simulink model "CHM2Ctrl_Caller"  (R2018b)
settings: Solver=FixedStepDiscrete  StartTime=0.0  StopTime=10.0  FixedStep=0.01  RelTol=1e-3
undefined symbols (not defined in the file or in its folder): CHM2ActiveReqChk_Cal, CHM2ActiveSubStateCtrl_Cal, CHM2StateCtrl_Cal, KeSMSbMdChime2Enable_Val
settings Model: Creator=sn2xws  LastModifiedBy=sn2xws
settings DataIOCC: SaveFormat=StructureWithTime
settings OptimizationCC: DefaultParameterBehavior=Inlined  EnhancedBackFolding=on  PassReuseOutputArgsAs=Individual arguments  ZeroExternalMemoryAtStartup=off  ZeroInternalMemoryAtStartup=off  OptimizeBlockOrder=speed  DifferentSizesBufferReuse=on  OptimizationCustomize=off
settings DebuggingCC: ParameterTunabilityLossMsg=error
settings SFSimCC: MATLABDynamicMemAlloc=off
settings RTWCC: SystemTargetFile=autosar.tlc  GenCodeOnly=on  TemplateMakefile=ert_default_tmf  Description=AUTOSAR  GenerateReport=on  IncludeHyperlinkInReport=on  LaunchReport=on  GenerateTraceInfo=on  GenerateTraceReport=on  GenerateTraceReportSl=on  GenerateTraceReportSf=on  GenerateTraceReportEml=on  GenerateCodeMetricsReport=on
settings CodeAppCC: ForceParamTrailComments=on  IgnoreCustomStorageClasses=off  OperatorAnnotations=on  SimulinkDataObjDesc=on  SFDataObjDesc=on  InsertBlockDesc=on
settings STFCustomTargetCC: TargetLangStandard=C99 (ISO)  MultiwordLength=256  ParMdlRefBuildCompliant=on  CompOptLevelCompliant=on  IncludeMdlTerminateFcn=off  CombineOutputUpdateFcns=on  SuppressErrorStatus=on  ERTCustomFileBanners=on  SupportNonFinite=off  SupportComplex=off  SupportContinuousTime=off  SupportNonInlinedSFcns=off  RemoveResetFunc=on  MATLABClassNameForMDSCustomization=Simulink.SoftwareTarget.ERTCustomization  AutosarCompliant=on  UseToolchainInfoCompliant=on  LookupTableObjectStructAxisOrder=2,1,3,4,...  LUTObjectStructOrderEvenSpacing=Size,Table,Breakpoints  SystemTargetFile=autosar.tlc
settings ERTTargetCC: TargetLangStandard=C99 (ISO)  ConcurrentExecutionCompliant=off  IncludeMdlTerminateFcn=off  SuppressErrorStatus=on  SupportNonFinite=off  SupportComplex=off  ModelStepFunctionPrototypeControlCompliant=off  CPPClassGenCompliant=off  AutosarCompliant=on  LookupTableObjectStructAxisOrder=2,1,3,4,...  LUTObjectStructOrderEvenSpacing=Size,Table,Breakpoints  InlinedParameterPlacement=NonHierarchical  ERTCustomFileTemplate=example_file_process.tlc  ERTFilePackagingFormat=Compact

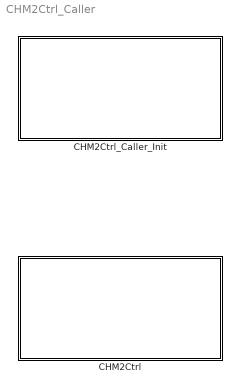
== system CHM2Ctrl_Caller ==
  CHM2Ctrl : Subsystem
  CHM2Ctrl_Caller_Init : Subsystem

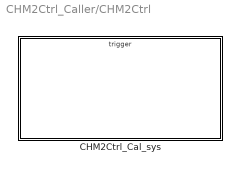
== system CHM2Ctrl_Caller/CHM2Ctrl ==
  CHM2Ctrl_Cal_sys : Subsystem

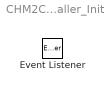
== system CHM2Ctrl_Caller/CHM2Ctrl_Caller_Init ==
  Event Listener : EventListener  EventName=reset

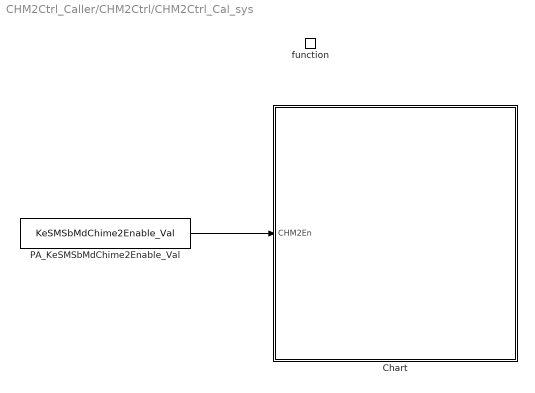
== system CHM2Ctrl_Caller/CHM2Ctrl/CHM2Ctrl_Cal_sys ==
  function : TriggerPort  TriggerType=function-call  IsSimulinkFunction=on  FunctionName=CHM2Ctrl_Cal  VariantControl=(inherit)
  Chart : Stateflow chart  TreatAsAtomicUnit=on
  PA_KeSMSbMdChime2Enable_Val : Constant  Value=KeSMSbMdChime2Enable_Val
  wires:
  PA_KeSMSbMdChime2Enable_Val/1 -> Chart/1(CHM2En)

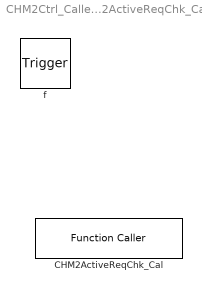
== system CHM2Ctrl_Caller/CHM2Ctrl/CHM2Ctrl_Cal_sys/Chart/CHM2ActiveReqChk_Cal ==
  f : TriggerPort  TriggerType=function-call  VariantControl=(inherit)
      settings: CopyFcn=Stateflow.SLINSF.SimulinkMan.removeBlockPreDeleteFcn  PreDeleteFcn=Stateflow.SLINSF.SimulinkMan.unsafePredeleteFcn
  CHM2ActiveReqChk_Cal : FunctionCaller  FunctionPrototype=CHM2ActiveReqChk_Cal()

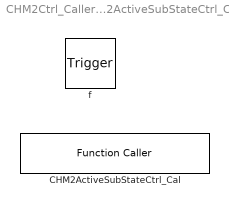
== system CHM2Ctrl_Caller/CHM2Ctrl/CHM2Ctrl_Cal_sys/Chart/CHM2ActiveSubStateCtrl_Cal ==
  f : TriggerPort  TriggerType=function-call  VariantControl=(inherit)
      settings: CopyFcn=Stateflow.SLINSF.SimulinkMan.removeBlockPreDeleteFcn  PreDeleteFcn=Stateflow.SLINSF.SimulinkMan.unsafePredeleteFcn
  CHM2ActiveSubStateCtrl_Cal : FunctionCaller  FunctionPrototype=CHM2ActiveSubStateCtrl_Cal()

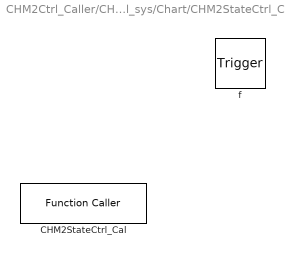
== system CHM2Ctrl_Caller/CHM2Ctrl/CHM2Ctrl_Cal_sys/Chart/CHM2StateCtrl_Cal ==
  f : TriggerPort  TriggerType=function-call  VariantControl=(inherit)
      settings: CopyFcn=Stateflow.SLINSF.SimulinkMan.removeBlockPreDeleteFcn  PreDeleteFcn=Stateflow.SLINSF.SimulinkMan.unsafePredeleteFcn
  CHM2StateCtrl_Cal : FunctionCaller  FunctionPrototype=CHM2StateCtrl_Cal()

== stateflow chart CHM2Ctrl_Caller/CHM2Ctrl/CHM2Ctrl_Cal_sys/Chart ==
  state CHM2ActiveReqChk_Cal [function]
  state CHM2ActiveSubStateCtrl_Cal [function]
  state CHM2StateCtrl_Cal [function]
  (default) -> (junction 2)
  (junction 2) -> (junction 9) [order 1] : [!CHM2En]
  (junction 2) -> (junction 4) [order 2] : {
      | CHM2ActiveReqChk_Cal();
      | CHM2StateCtrl_Cal();
      | CHM2ActiveSubStateCtrl_Cal();
      | }
  (junction 9) -> (junction 11)
  (junction 11) -> (junction 4)
  (junction 4) -> (junction 14)
  data: CHM2En input
